simulink model "mass_sim"  (R2016b)
settings: Solver=ode45  StartTime=0.0  StopTime=60  RelTol=1e-3  EnableMultiTasking=on
InitFcn:
  | addpath ./..
  | mass_param
  | massParamHWf
values from neighbouring files (symbols this model uses):
  K_leadlag = 65    [massParamHWf.m]
undefined symbols (not defined in the file or in its folder): dD_leadlag, nD_leadlag, P
settings Model: Creator=beard  LastModifiedBy=mclain
settings DataIOCC: LimitDataPoints=on  SaveFormat=Array  SignalLoggingSaveFormat=ModelDataLogs
settings OptimizationCC: ExpressionDepthLimit=2147483647  InitFltsAndDblsToZero=on  LifeSpan=inf
settings DebuggingCC: UnderspecifiedInitializationDetection=Classic  MergeDetectMultiDrivingBlocksExec=none  SolverPrmCheckMsg=warning  FcnCallInpInsideContextMsg=warning  StateNameClashWarn=warning  SFUnexpectedBacktrackingDiag=warning  SFNoUnconditionalDefaultTransitionDiag=warning  SFExecutionAtInitializationDiag=none
settings HardwareCC: ProdBitPerPointer=32  ProdBitPerSizeT=32  ProdBitPerPtrDiffT=32  ProdLargestAtomicFloat=None  ProdIntDivRoundTo=Undefined  ProdEndianess=Unspecified  ProdWordSize=32  ProdHWDeviceType=32-bit Generic
settings ModelReferenceCC: PropagateSignalLabelsOutOfModel=off
settings GRTTargetCC: TargetLangStandard=C89/C90 (ANSI)  GeneratePreprocessorConditionals=Disable all  CombineOutputUpdateFcns=off  GRTInterface=on
settings ConfigComp: CovMetricSettings=dw  CovHtmlReporting=on  CovSaveCumulativeToWorkspaceVar=on  CovSaveSingleToWorkspaceVar=on  CovExternalEMLEnable=off

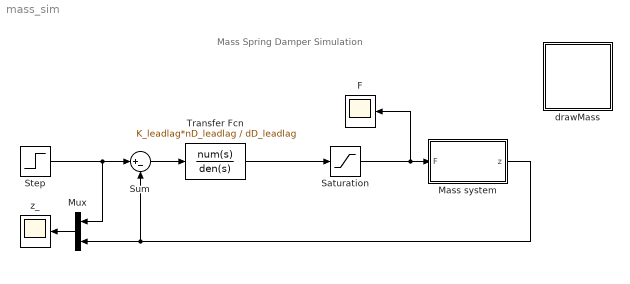
== system mass_sim ==
  note: Mass Spring Damper Simulation
  F : Scope
  Mass system : Subsystem
  Mux : Mux  Inputs=2
  Saturation : Saturate  UpperLimit=P.F_max  LowerLimit=-P.F_max
  Step : Step  SampleTime=0
  Sum : Sum  Inputs=|+-
  Transfer Fcn : TransferFcn  Numerator=K_leadlag*nD_leadlag  Denominator=dD_leadlag
  drawMass : Subsystem
      mask Display: image(imread('tv.jpg'))
  z_ : Scope
  wires:
  Mux/1 -> z_/1
  Step/1 -> Sum/1, Mux/1
  Transfer Fcn/1 -> Saturation/1
  Mass system/1(z) -> Mux/2, Sum/2
  Saturation/1 -> Mass system/1(F), F/1
  Sum/1 -> Transfer Fcn/1

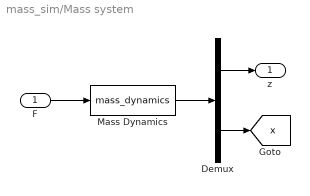
== system mass_sim/Mass system ==
  F : Inport
  Demux : Demux  Outputs=[1;2]
  Mass Dynamics : S-Function  FunctionName=mass_dynamics  Parameters=P  SFunctionDeploymentMode=off  EnableBusSupport=off
  z : Outport
  tag scope: x=global
  wires:
  F/1 -> Mass Dynamics/1
  Mass Dynamics/1 -> Demux/1
  Demux/1 -> z/1
  Demux/2 -> [x]

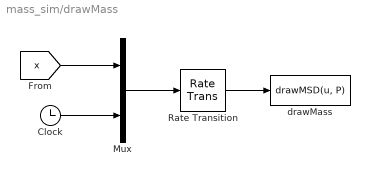
== system mass_sim/drawMass ==
  Clock : Clock
  Mux : Mux  Inputs=2
  Rate Transition : RateTransition  OutPortSampleTime=P.t_plot
  drawMass : MATLABFcn  MATLABFcn=drawMSD(u, P)  OutputDimensions=0
  wires:
  Mux/1 -> Rate Transition/1
  [x] -> Mux/1
  Clock/1 -> Mux/2
  Rate Transition/1 -> drawMass/1
